simulink model "SIMULINK_PID_Tracking"  (R2023b)
settings: Solver=FixedStepAuto  StartTime=0.0  StopTime=sim_end_time  FixedStep=fixed_step_size  RelTol=1e-3
undefined symbols (not defined in the file): a, act_end, b, battery_threshold, bb, draw_gif, droneyeeUAV2_NUM, droneyeeUAV3_NUM, droneyeeUAV4_NUM, droneyeeUAV5_NUM, fixed_step_size, k, KD_x, KD_y, kd_z, KDD_x, KDD_y, KI_x, KI_y, ki_z, KII_x, KII_y, KP_x, KP_y, kp_z, KPP_x, KPP_y, lmt, omega, R, sim_end_time, uav10num, uav1num, uav2num, uav3num, uav4num, uav5num, uav6num, uav7num, uav8num, uav9num, UAV_NUM, Vel_Switch_1, Vel_Switch_10, Vel_Switch_11, Vel_Switch_12, Vel_Switch_13, Vel_Switch_14, Vel_Switch_15, Vel_Switch_16, Vel_Switch_17, Vel_Switch_18, Vel_Switch_19, Vel_Switch_2, Vel_Switch_20, Vel_Switch_3, Vel_Switch_4, Vel_Switch_5, Vel_Switch_6, Vel_Switch_7 ... (+12)
libraries: simulink x120, aerolibanimutils x1
(part 6 of 10)

== system SIMULINK_PID_Tracking/send_ctrl_signal_UAV/Send Command 2 ==
  pos : Inport
  u : Inport  Port=2
  Bus Selector : BusSelector  OutputSignals=droneyeeUAV2_states.x,droneyeeUAV2_states.y  OutputAsBus=on
  Bus Selector1 : BusSelector  OutputSignals=uav2.u_vx,uav2.u_vy,uav2.u_vz,uav2.u_rate_roll,uav2.u_rate_pitch,uav2.u_rate_yaw
  Clock : Clock
  Compare To Constant : simulink/Logic and Bit Operations/Compare To Constant  relop=>=  const=0.1  OutDataTypeStr=boolean
  Constant : Constant  Value=sim_end_time
  Constant1 : Constant  Value=0
  Constant2 : Constant  Value=droneyeeUAV2_NUM
  Constant3 : Constant  Value=Vel_Switch_2
  Constant4 : Constant  Value=0
  K : Gain
  K1 : Gain
  K2 : Gain
  Logical Operator : Logic  Inputs=3  AllPortsSameDT=off  OutDataTypeStr=boolean
  Mux : Mux  Inputs=8
  Mux1 : Mux  Inputs=5
  Subsystem : Subsystem
  Sum : Sum  Inputs=|-+
  Switch{1..3,6,12} (5 alike) : Switch  Criteria=u2 > Threshold  Threshold=0.001  SaturateOnIntegerOverflow=off  InputSameDT=off
  Switch4 : Switch  Criteria=u2 > Threshold  SaturateOnIntegerOverflow=off  InputSameDT=off
  Switch5 : Switch  Criteria=u2 > Threshold  SaturateOnIntegerOverflow=off  InputSameDT=off
  uav2 : Constant
  tag scope: copterSend2=global, sim_CopterSend2=global
  wires:
  Constant1/1 -> Switch3/3, Switch2/3, Switch1/3, Switch12/3
  Switch1/1 -> K/1
  Bus Selector1/2 -> Switch1/1  "<u_vy>"
  Switch2/1 -> K2/1
  Bus Selector1/3 -> Switch2/1  "<u_vz>"
  Switch3/1 -> K1/1
  Logical Operator/1 -> Switch1/2, Switch12/2, Switch2/2, Switch3/2
  Clock/1 -> Sum/1
  Constant/1 -> Sum/2
  Sum/1 -> Compare To Constant/1
  Compare To Constant/1 -> Logical Operator/2
  pos/1 -> Bus Selector/1
  Bus Selector/1 -> Subsystem/1(In1)
  u/1 -> Bus Selector1/1
  Bus Selector1/1 -> Switch12/1  "<u_vx>"
  Bus Selector1/6 -> Switch3/1  "<u_rate_yaw>"
  Bus Selector1/4 -> Mux/5  "<u_rate_roll>"
  Bus Selector1/5 -> Mux/6  "<u_rate_pitch>"
  Constant2/1 -> Mux/1
  Constant3/1 -> Logical Operator/3
  Switch6/1 -> Mux/8
  Subsystem/1(Out1) -> Logical Operator/1
  Switch4/1 -> [sim_CopterSend2]
  [sim_flag] -> Switch5/2, Switch4/2
  Switch5/1 -> [copterSend2]
  Mux/1 -> Switch5/1
  Mux1/1 -> Switch4/3
  K/1 -> Mux1/3, Mux/3
  K1/1 -> Mux1/5, Mux/7
  K2/1 -> Mux1/4, Mux/4
  Switch12/1 -> Mux1/2, Mux/2
  Constant4/1 -> Mux1/1
  uav2/1 -> Switch6/3
  [mode1] -> Switch6/2, Switch6/1

== system SIMULINK_PID_Tracking/send_ctrl_signal_UAV/Send Command 3 ==
  pos : Inport
  u : Inport  Port=2
  Bus Selector : BusSelector  OutputSignals=droneyeeUAV3_states.x,droneyeeUAV3_states.y  OutputAsBus=on
  Bus Selector1 : BusSelector  OutputSignals=uav3.u_vx,uav3.u_vy,uav3.u_vz,uav3.u_rate_roll,uav3.u_rate_pitch,uav3.u_rate_yaw
  Clock : Clock
  Compare To Constant : simulink/Logic and Bit Operations/Compare To Constant  relop=>=  const=0.1  OutDataTypeStr=boolean
  Constant : Constant  Value=sim_end_time
  Constant1 : Constant  Value=0
  Constant2 : Constant  Value=droneyeeUAV3_NUM
  Constant3 : Constant  Value=Vel_Switch_3
  Constant4 : Constant  Value=0
  K : Gain
  K1 : Gain
  K2 : Gain
  Logical Operator : Logic  Inputs=3  AllPortsSameDT=off  OutDataTypeStr=boolean
  Mux : Mux  Inputs=8
  Mux1 : Mux  Inputs=5
  Subsystem : Subsystem
  Sum : Sum  Inputs=|-+
  Switch{1..3,6,12} (5 alike) : Switch  Criteria=u2 > Threshold  Threshold=0.001  SaturateOnIntegerOverflow=off  InputSameDT=off
  Switch4 : Switch  Criteria=u2 > Threshold  SaturateOnIntegerOverflow=off  InputSameDT=off
  Switch5 : Switch  Criteria=u2 > Threshold  SaturateOnIntegerOverflow=off  InputSameDT=off
  uav3 : Constant
  tag scope: copterSend3=global, sim_CopterSend3=global
  wires:
  Constant1/1 -> Switch3/3, Switch2/3, Switch1/3, Switch12/3
  Switch1/1 -> K/1
  Bus Selector1/2 -> Switch1/1  "<u_vy>"
  Switch2/1 -> K2/1
  Bus Selector1/3 -> Switch2/1  "<u_vz>"
  Switch3/1 -> K1/1
  Logical Operator/1 -> Switch1/2, Switch12/2, Switch2/2, Switch3/2
  Clock/1 -> Sum/1
  Constant/1 -> Sum/2
  Sum/1 -> Compare To Constant/1
  Compare To Constant/1 -> Logical Operator/2
  pos/1 -> Bus Selector/1
  Bus Selector/1 -> Subsystem/1(In1)
  u/1 -> Bus Selector1/1
  Bus Selector1/1 -> Switch12/1  "<u_vx>"
  Bus Selector1/6 -> Switch3/1  "<u_rate_yaw>"
  Bus Selector1/4 -> Mux/5  "<u_rate_roll>"
  Bus Selector1/5 -> Mux/6  "<u_rate_pitch>"
  Constant2/1 -> Mux/1
  Constant3/1 -> Logical Operator/3
  Switch6/1 -> Mux/8
  Subsystem/1(Out1) -> Logical Operator/1
  Switch4/1 -> [sim_CopterSend3]
  [sim_flag] -> Switch5/2, Switch4/2
  Switch5/1 -> [copterSend3]
  Mux/1 -> Switch5/1
  Mux1/1 -> Switch4/3
  K/1 -> Mux1/3, Mux/3
  K1/1 -> Mux1/5, Mux/7
  K2/1 -> Mux1/4, Mux/4
  Switch12/1 -> Mux1/2, Mux/2
  Constant4/1 -> Mux1/1
  uav3/1 -> Switch6/3
  [mode1] -> Switch6/2, Switch6/1

== system SIMULINK_PID_Tracking/send_ctrl_signal_UAV/Send Command 4 ==
  pos : Inport
  u : Inport  Port=2
  Bus Selector : BusSelector  OutputSignals=droneyeeUAV4_states.x,droneyeeUAV4_states.y  OutputAsBus=on
  Bus Selector1 : BusSelector  OutputSignals=uav4.u_vx,uav4.u_vy,uav4.u_vz,uav4.u_rate_roll,uav4.u_rate_pitch,uav4.u_rate_yaw
  Clock : Clock
  Compare To Constant : simulink/Logic and Bit Operations/Compare To Constant  relop=>=  const=0.1  OutDataTypeStr=boolean
  Constant : Constant  Value=sim_end_time
  Constant1 : Constant  Value=0
  Constant2 : Constant  Value=droneyeeUAV4_NUM
  Constant3 : Constant  Value=Vel_Switch_4
  Constant4 : Constant  Value=0
  K : Gain
  K1 : Gain
  K2 : Gain
  Logical Operator : Logic  Inputs=3  AllPortsSameDT=off  OutDataTypeStr=boolean
  Mux : Mux  Inputs=8
  Mux1 : Mux  Inputs=5
  Subsystem : Subsystem
  Sum : Sum  Inputs=|-+
  Switch{1..3,6,12} (5 alike) : Switch  Criteria=u2 > Threshold  Threshold=0.001  SaturateOnIntegerOverflow=off  InputSameDT=off
  Switch4 : Switch  Criteria=u2 > Threshold  SaturateOnIntegerOverflow=off  InputSameDT=off
  Switch5 : Switch  Criteria=u2 > Threshold  SaturateOnIntegerOverflow=off  InputSameDT=off
  uav4 : Constant
  tag scope: copterSend4=global, sim_CopterSend4=global
  wires:
  Constant1/1 -> Switch3/3, Switch2/3, Switch1/3, Switch12/3
  Switch1/1 -> K/1
  Bus Selector1/2 -> Switch1/1  "<u_vy>"
  Switch2/1 -> K2/1
  Bus Selector1/3 -> Switch2/1  "<u_vz>"
  Switch3/1 -> K1/1
  Logical Operator/1 -> Switch1/2, Switch12/2, Switch2/2, Switch3/2
  Clock/1 -> Sum/1
  Constant/1 -> Sum/2
  Sum/1 -> Compare To Constant/1
  Compare To Constant/1 -> Logical Operator/2
  pos/1 -> Bus Selector/1
  u/1 -> Bus Selector1/1
  Bus Selector1/1 -> Switch12/1  "<u_vx>"
  Bus Selector1/6 -> Switch3/1  "<u_rate_yaw>"
  Bus Selector1/4 -> Mux/5  "<u_rate_roll>"
  Bus Selector1/5 -> Mux/6  "<u_rate_pitch>"
  Constant2/1 -> Mux/1
  Constant3/1 -> Logical Operator/3
  Switch6/1 -> Mux/8
  Bus Selector/1 -> Subsystem/1(In1)
  Subsystem/1(Out1) -> Logical Operator/1
  Switch4/1 -> [sim_CopterSend4]
  [sim_flag] -> Switch5/2, Switch4/2
  Switch5/1 -> [copterSend4]
  Mux/1 -> Switch5/1
  Mux1/1 -> Switch4/3
  K/1 -> Mux1/3, Mux/3
  K1/1 -> Mux1/5, Mux/7
  K2/1 -> Mux1/4, Mux/4
  Switch12/1 -> Mux1/2, Mux/2
  Constant4/1 -> Mux1/1
  uav4/1 -> Switch6/3
  [mode1] -> Switch6/2, Switch6/1

== system SIMULINK_PID_Tracking/send_ctrl_signal_UAV/Send Command 5 ==
  pos : Inport
  u : Inport  Port=2
  Bus Selector : BusSelector  OutputSignals=x,y  OutputAsBus=on
  Bus Selector1 : BusSelector  OutputSignals=u_vx,u_vy,u_vz,u_rate_roll,u_rate_pitch,u_rate_yaw
  Clock : Clock
  Compare To Constant : simulink/Logic and Bit Operations/Compare To Constant  relop=>=  const=0.1  OutDataTypeStr=boolean
  Constant : Constant  Value=sim_end_time
  Constant1 : Constant  Value=0
  Constant2 : Constant  Value=droneyeeUAV5_NUM
  Constant3 : Constant  Value=Vel_Switch_5
  Constant4 : Constant  Value=0
  K : Gain
  K1 : Gain
  K2 : Gain
  Logical Operator : Logic  Inputs=3  AllPortsSameDT=off  OutDataTypeStr=boolean
  Mux : Mux  Inputs=8
  Mux1 : Mux  Inputs=5
  Subsystem : Subsystem
  Sum : Sum  Inputs=|-+
  Switch{1..3,6,12} (5 alike) : Switch  Criteria=u2 > Threshold  Threshold=0.001  SaturateOnIntegerOverflow=off  InputSameDT=off
  Switch4 : Switch  Criteria=u2 > Threshold  SaturateOnIntegerOverflow=off  InputSameDT=off
  Switch5 : Switch  Criteria=u2 > Threshold  SaturateOnIntegerOverflow=off  InputSameDT=off
  uav5 : Constant
  tag scope: copterSend5=global, sim_CopterSend5=global
  wires:
  Constant1/1 -> Switch3/3, Switch2/3, Switch1/3, Switch12/3
  Switch1/1 -> K/1
  Bus Selector1/2 -> Switch1/1  "<u_vy>"
  Switch2/1 -> K2/1
  Bus Selector1/3 -> Switch2/1  "<u_vz>"
  Switch3/1 -> K1/1
  Logical Operator/1 -> Switch1/2, Switch12/2, Switch2/2, Switch3/2
  Clock/1 -> Sum/1
  Constant/1 -> Sum/2
  Sum/1 -> Compare To Constant/1
  Compare To Constant/1 -> Logical Operator/2
  pos/1 -> Bus Selector/1
  Bus Selector/1 -> Subsystem/1(In1)
  u/1 -> Bus Selector1/1
  Bus Selector1/1 -> Switch12/1  "<u_vx>"
  Bus Selector1/6 -> Switch3/1  "<u_rate_yaw>"
  Bus Selector1/4 -> Mux/5  "<u_rate_roll>"
  Bus Selector1/5 -> Mux/6  "<u_rate_pitch>"
  Subsystem/1(Out1) -> Logical Operator/1
  Constant2/1 -> Mux/1
  Constant3/1 -> Logical Operator/3
  Switch6/1 -> Mux/8
  Switch4/1 -> [sim_CopterSend5]
  [sim_flag] -> Switch5/2, Switch4/2
  Switch5/1 -> [copterSend5]
  Mux/1 -> Switch5/1
  Mux1/1 -> Switch4/3
  K/1 -> Mux1/3, Mux/3
  K1/1 -> Mux1/5, Mux/7
  K2/1 -> Mux1/4, Mux/4
  Switch12/1 -> Mux1/2, Mux/2
  Constant4/1 -> Mux1/1
  uav5/1 -> Switch6/3
  [mode1] -> Switch6/2, Switch6/1

== system SIMULINK_PID_Tracking/send_ctrl_signal_UAV/Send Command 6 ==
  pos : Inport
  u : Inport  Port=2
  Bus Selector : BusSelector  OutputSignals=x,y  OutputAsBus=on
  Bus Selector1 : BusSelector  OutputSignals=u_vx,u_vy,u_vz,u_rate_roll,u_rate_pitch,u_rate_yaw
  Clock : Clock
  Compare To Constant : simulink/Logic and Bit Operations/Compare To Constant  relop=>=  const=0.1  OutDataTypeStr=boolean
  Constant : Constant  Value=sim_end_time
  Constant1 : Constant  Value=0
  Constant2 : Constant  Value=uav6num
  Constant3 : Constant  Value=Vel_Switch_6
  Constant4 : Constant  Value=0
  K : Gain
  K1 : Gain
  K2 : Gain
  Logical Operator : Logic  Inputs=3  AllPortsSameDT=off  OutDataTypeStr=boolean
  Mux : Mux  Inputs=8
  Mux1 : Mux  Inputs=5
  Subsystem : Subsystem
  Sum : Sum  Inputs=|-+
  Switch{1..3,6,12} (5 alike) : Switch  Criteria=u2 > Threshold  Threshold=0.001  SaturateOnIntegerOverflow=off  InputSameDT=off
  Switch4 : Switch  Criteria=u2 > Threshold  SaturateOnIntegerOverflow=off  InputSameDT=off
  Switch5 : Switch  Criteria=u2 > Threshold  SaturateOnIntegerOverflow=off  InputSameDT=off
  uav6 : Constant  Value=0
  tag scope: copterSend6=global, sim_CopterSend6=global
  wires:
  Constant1/1 -> Switch3/3, Switch2/3, Switch1/3, Switch12/3
  K1/1 -> Mux1/5, Mux/7
  Switch1/1 -> K/1
  Bus Selector1/2 -> Switch1/1  "<u_vy>"
  Switch2/1 -> K2/1
  Bus Selector1/3 -> Switch2/1  "<u_vz>"
  Switch3/1 -> K1/1
  Logical Operator/1 -> Switch1/2, Switch12/2, Switch2/2, Switch3/2
  K2/1 -> Mux1/4, Mux/4
  Clock/1 -> Sum/1
  Constant/1 -> Sum/2
  Sum/1 -> Compare To Constant/1
  Compare To Constant/1 -> Logical Operator/2
  pos/1 -> Bus Selector/1
  Bus Selector/1 -> Subsystem/1(In1)
  u/1 -> Bus Selector1/1
  Bus Selector1/1 -> Switch12/1  "<u_vx>"
  Bus Selector1/6 -> Switch3/1  "<u_rate_yaw>"
  Bus Selector1/4 -> Mux/5  "<u_rate_roll>"
  Bus Selector1/5 -> Mux/6  "<u_rate_pitch>"
  Constant2/1 -> Mux/1
  Constant3/1 -> Logical Operator/3
  Switch12/1 -> Mux1/2, Mux/2
  K/1 -> Mux1/3, Mux/3
  Switch6/1 -> Mux/8
  Subsystem/1(Out1) -> Logical Operator/1
  Constant4/1 -> Mux1/1
  Switch4/1 -> [sim_CopterSend6]
  Mux1/1 -> Switch4/3
  Mux/1 -> Switch5/1
  Switch5/1 -> [copterSend6]
  [sim_flag] -> Switch5/2, Switch4/2
  uav6/1 -> Switch6/3
  [mode1] -> Switch6/2, Switch6/1

== system SIMULINK_PID_Tracking/send_ctrl_signal_UAV/Send Command 7 ==
  pos : Inport
  u : Inport  Port=2
  Bus Selector : BusSelector  OutputSignals=x,y  OutputAsBus=on
  Bus Selector1 : BusSelector  OutputSignals=u_vx,u_vy,u_vz,u_rate_roll,u_rate_pitch,u_rate_yaw
  Clock : Clock
  Compare To Constant : simulink/Logic and Bit Operations/Compare To Constant  relop=>=  const=0.1  OutDataTypeStr=boolean
  Constant : Constant  Value=sim_end_time
  Constant1 : Constant  Value=0
  Constant2 : Constant  Value=uav7num
  Constant3 : Constant  Value=Vel_Switch_7
  Constant4 : Constant  Value=0
  K : Gain
  K1 : Gain
  K2 : Gain
  Logical Operator : Logic  Inputs=3  AllPortsSameDT=off  OutDataTypeStr=boolean
  Mux : Mux  Inputs=8
  Mux1 : Mux  Inputs=5
  Subsystem : Subsystem
  Sum : Sum  Inputs=|-+
  Switch{1..3,6,12} (5 alike) : Switch  Criteria=u2 > Threshold  Threshold=0.001  SaturateOnIntegerOverflow=off  InputSameDT=off
  Switch4 : Switch  Criteria=u2 > Threshold  SaturateOnIntegerOverflow=off  InputSameDT=off
  Switch5 : Switch  Criteria=u2 > Threshold  SaturateOnIntegerOverflow=off  InputSameDT=off
  uav7 : Constant  Value=0
  tag scope: copterSend7=global, sim_CopterSend7=global
  wires:
  Constant1/1 -> Switch3/3, Switch2/3, Switch1/3, Switch12/3
  K1/1 -> Mux1/5, Mux/7
  Switch1/1 -> K/1
  Bus Selector1/2 -> Switch1/1  "<u_vy>"
  Switch2/1 -> K2/1
  Bus Selector1/3 -> Switch2/1  "<u_vz>"
  Switch3/1 -> K1/1
  Logical Operator/1 -> Switch1/2, Switch12/2, Switch2/2, Switch3/2
  K2/1 -> Mux1/4, Mux/4
  Clock/1 -> Sum/1
  Constant/1 -> Sum/2
  Sum/1 -> Compare To Constant/1
  Compare To Constant/1 -> Logical Operator/2
  pos/1 -> Bus Selector/1
  Bus Selector/1 -> Subsystem/1(In1)
  u/1 -> Bus Selector1/1
  Bus Selector1/1 -> Switch12/1  "<u_vx>"
  Bus Selector1/6 -> Switch3/1  "<u_rate_yaw>"
  Bus Selector1/4 -> Mux/5  "<u_rate_roll>"
  Bus Selector1/5 -> Mux/6  "<u_rate_pitch>"
  Constant2/1 -> Mux/1
  Constant3/1 -> Logical Operator/3
  Switch12/1 -> Mux1/2, Mux/2
  K/1 -> Mux1/3, Mux/3
  Switch6/1 -> Mux/8
  Subsystem/1(Out1) -> Logical Operator/1
  Constant4/1 -> Mux1/1
  Switch4/1 -> [sim_CopterSend7]
  Mux1/1 -> Switch4/3
  Mux/1 -> Switch5/1
  Switch5/1 -> [copterSend7]
  [sim_flag] -> Switch5/2, Switch4/2
  uav7/1 -> Switch6/3
  [mode1] -> Switch6/2, Switch6/1

== system SIMULINK_PID_Tracking/send_ctrl_signal_UAV/Send Command 8 ==
  pos : Inport
  u : Inport  Port=2
  Bus Selector : BusSelector  OutputSignals=x,y  OutputAsBus=on
  Bus Selector1 : BusSelector  OutputSignals=u_vx,u_vy,u_vz,u_rate_roll,u_rate_pitch,u_rate_yaw
  Clock : Clock
  Compare To Constant : simulink/Logic and Bit Operations/Compare To Constant  relop=>=  const=0.1  OutDataTypeStr=boolean
  Constant : Constant  Value=sim_end_time
  Constant1 : Constant  Value=0
  Constant2 : Constant  Value=uav8num
  Constant3 : Constant  Value=Vel_Switch_8
  Constant4 : Constant  Value=0
  K : Gain
  K1 : Gain
  K2 : Gain
  Logical Operator : Logic  Inputs=3  AllPortsSameDT=off  OutDataTypeStr=boolean
  Mux : Mux  Inputs=8
  Mux1 : Mux  Inputs=5
  Subsystem : Subsystem
  Sum : Sum  Inputs=|-+
  Switch{1..3,6,12} (5 alike) : Switch  Criteria=u2 > Threshold  Threshold=0.001  SaturateOnIntegerOverflow=off  InputSameDT=off
  Switch4 : Switch  Criteria=u2 > Threshold  SaturateOnIntegerOverflow=off  InputSameDT=off
  Switch5 : Switch  Criteria=u2 > Threshold  SaturateOnIntegerOverflow=off  InputSameDT=off
  uav8 : Constant
  tag scope: copterSend8=global, sim_CopterSend8=global
  wires:
  Constant1/1 -> Switch3/3, Switch2/3, Switch1/3, Switch12/3
  K1/1 -> Mux1/5, Mux/7
  Switch1/1 -> K/1
  Bus Selector1/2 -> Switch1/1  "<u_vy>"
  Switch2/1 -> K2/1
  Bus Selector1/3 -> Switch2/1  "<u_vz>"
  Switch3/1 -> K1/1
  Logical Operator/1 -> Switch1/2, Switch12/2, Switch2/2, Switch3/2
  K2/1 -> Mux1/4, Mux/4
  Clock/1 -> Sum/1
  Constant/1 -> Sum/2
  Sum/1 -> Compare To Constant/1
  Compare To Constant/1 -> Logical Operator/2
  pos/1 -> Bus Selector/1
  Bus Selector/1 -> Subsystem/1(In1)
  u/1 -> Bus Selector1/1
  Bus Selector1/1 -> Switch12/1  "<u_vx>"
  Bus Selector1/6 -> Switch3/1  "<u_rate_yaw>"
  Bus Selector1/4 -> Mux/5  "<u_rate_roll>"
  Bus Selector1/5 -> Mux/6  "<u_rate_pitch>"
  Constant2/1 -> Mux/1
  Constant3/1 -> Logical Operator/3
  Switch12/1 -> Mux1/2, Mux/2
  K/1 -> Mux1/3, Mux/3
  Switch6/1 -> Mux/8
  Subsystem/1(Out1) -> Logical Operator/1
  Constant4/1 -> Mux1/1
  Switch4/1 -> [sim_CopterSend8]
  Mux1/1 -> Switch4/3
  Mux/1 -> Switch5/1
  Switch5/1 -> [copterSend8]
  [sim_flag] -> Switch5/2, Switch4/2
  uav8/1 -> Switch6/3
  [mode1] -> Switch6/2, Switch6/1

== system SIMULINK_PID_Tracking/send_ctrl_signal_UAV/Send Command 9 ==
  pos : Inport
  u : Inport  Port=2
  Bus Selector : BusSelector  OutputSignals=x,y  OutputAsBus=on
  Bus Selector1 : BusSelector  OutputSignals=u_vx,u_vy,u_vz,u_rate_roll,u_rate_pitch,u_rate_yaw
  Clock : Clock
  Compare To Constant : simulink/Logic and Bit Operations/Compare To Constant  relop=>=  const=0.1  OutDataTypeStr=boolean
  Constant : Constant  Value=sim_end_time
  Constant1 : Constant  Value=0
  Constant2 : Constant  Value=uav9num
  Constant3 : Constant  Value=Vel_Switch_9
  Constant4 : Constant  Value=0
  K : Gain
  K1 : Gain
  K2 : Gain
  Logical Operator : Logic  Inputs=3  AllPortsSameDT=off  OutDataTypeStr=boolean
  Mux : Mux  Inputs=8
  Mux1 : Mux  Inputs=5
  Subsystem : Subsystem
  Sum : Sum  Inputs=|-+
  Switch{1..3,6,12} (5 alike) : Switch  Criteria=u2 > Threshold  Threshold=0.001  SaturateOnIntegerOverflow=off  InputSameDT=off
  Switch4 : Switch  Criteria=u2 > Threshold  SaturateOnIntegerOverflow=off  InputSameDT=off
  Switch5 : Switch  Criteria=u2 > Threshold  SaturateOnIntegerOverflow=off  InputSameDT=off
  uav9 : Constant
  tag scope: copterSend9=global, sim_CopterSend9=global
  wires:
  Constant1/1 -> Switch3/3, Switch2/3, Switch1/3, Switch12/3
  K1/1 -> Mux1/5, Mux/7
  Switch1/1 -> K/1
  Bus Selector1/2 -> Switch1/1  "<u_vy>"
  Switch2/1 -> K2/1
  Bus Selector1/3 -> Switch2/1  "<u_vz>"
  Switch3/1 -> K1/1
  Logical Operator/1 -> Switch1/2, Switch12/2, Switch2/2, Switch3/2
  K2/1 -> Mux1/4, Mux/4
  Clock/1 -> Sum/1
  Constant/1 -> Sum/2
  Sum/1 -> Compare To Constant/1
  Compare To Constant/1 -> Logical Operator/2
  pos/1 -> Bus Selector/1
  Bus Selector/1 -> Subsystem/1(In1)
  u/1 -> Bus Selector1/1
  Bus Selector1/1 -> Switch12/1  "<u_vx>"
  Bus Selector1/6 -> Switch3/1  "<u_rate_yaw>"
  Bus Selector1/4 -> Mux/5  "<u_rate_roll>"
  Bus Selector1/5 -> Mux/6  "<u_rate_pitch>"
  Constant2/1 -> Mux/1
  Constant3/1 -> Logical Operator/3
  Switch12/1 -> Mux1/2, Mux/2
  K/1 -> Mux1/3, Mux/3
  Switch6/1 -> Mux/8
  Subsystem/1(Out1) -> Logical Operator/1
  Constant4/1 -> Mux1/1
  Switch4/1 -> [sim_CopterSend9]
  Mux1/1 -> Switch4/3
  Mux/1 -> Switch5/1
  Switch5/1 -> [copterSend9]
  [sim_flag] -> Switch5/2, Switch4/2
  uav9/1 -> Switch6/3
  [mode1] -> Switch6/2, Switch6/1

== system SIMULINK_PID_Tracking/send_ctrl_signal_UAV/Subsystem ==
  states_d : Inport
  ctrl : Inport  Port=2
  Bus Selector : BusSelector  OutputSignals=states1_2_d,states_3_4_d,states_5_6_d,states_7_8_d,states_9_10_d
  Bus Selector1 : BusSelector  OutputSignals=droneyeeUAV1_states,droneyeeUAV2_states  OutputAsBus=on
  Bus Selector2 : BusSelector  OutputSignals=ctrl_1_2,ctrl_3_4,ctrl_5_6,ctrl_7_8,ctrl_9_10
  Bus Selector5 : BusSelector  OutputSignals=droneyeeUAV9_states,droneyeeUAV10_states  OutputAsBus=on
  Bus Selector6 : BusSelector  OutputSignals=droneyeeUAV3_states,droneyeeUAV4_states  OutputAsBus=on
  Bus Selector7 : BusSelector  OutputSignals=droneyeeUAV5_states,droneyeeUAV6_states  OutputAsBus=on
  Bus Selector8 : BusSelector  OutputSignals=droneyeeUAV7_states,droneyeeUAV8_states  OutputAsBus=on
  logger_UAV : Subsystem
  wires:
  Bus Selector/1 -> logger_UAV/6(state_d1_2)  "<states1_2_d>"
  Bus Selector/2 -> logger_UAV/7(state_d3_4)  "<states_3_4_d>"
  [uav_states] -> Bus Selector8/1, Bus Selector7/1, Bus Selector6/1, Bus Selector1/1, Bus Selector5/1
  Bus Selector1/1 -> logger_UAV/1(state1_2)
  Bus Selector6/1 -> logger_UAV/2(state3_4)
  Bus Selector2/2 -> logger_UAV/12(u3_4)  "<ctrl_3_4>"
  Bus Selector2/1 -> logger_UAV/11(u1_2)  "<ctrl_1_2>"
  Bus Selector7/1 -> logger_UAV/3(state5_6)
  Bus Selector2/3 -> logger_UAV/13(u5_6)  "<ctrl_5_6>"
  states_d/1 -> Bus Selector/1
  ctrl/1 -> Bus Selector2/1
  Bus Selector/3 -> logger_UAV/8(state_d5_6)  "<states_5_6_d>"
  Bus Selector8/1 -> logger_UAV/4(state7_8)
  Bus Selector5/1 -> logger_UAV/5(In5)
  Bus Selector/4 -> logger_UAV/9(In9)  "<states_7_8_d>"
  Bus Selector/5 -> logger_UAV/10(In10)  "<states_9_10_d>"
  Bus Selector2/4 -> logger_UAV/14(In14)  "<ctrl_7_8>"
  Bus Selector2/5 -> logger_UAV/15(In15)  "<ctrl_9_10>"

== system SIMULINK_PID_Tracking/send_ctrl_signal_car1/Send Command 1 ==
  pos : Inport
  u : Inport  Port=2
  Bus Selector : BusSelector  OutputSignals=droneyeeCAR1_states.x,droneyeeCAR1_states.y  OutputAsBus=on
  Bus Selector1 : BusSelector  OutputSignals=CAR1.u_vx,CAR1.u_vy,CAR1.u_vz,CAR1.u_rate_roll,CAR1.u_rate_pitch,CAR1.u_rate_yaw
  Clock : Clock
  Compare To Constant : simulink/Logic and Bit Operations/Compare To Constant  relop=>=  const=0.1  OutDataTypeStr=boolean
  Constant : Constant  Value=sim_end_time
  Constant1 : Constant  Value=0
  Constant2 : Constant  Value=uav1num
  Constant3 : Constant  Value=Vel_Switch_11
  Constant4 : Constant  Value=0
  K : Gain
  K1 : Gain
  K2 : Gain
  Logical Operator : Logic  Inputs=3  AllPortsSameDT=off  OutDataTypeStr=boolean
  Mux : Mux  Inputs=8
  Mux1 : Mux  Inputs=5
  Subsystem : Subsystem
  Sum : Sum  Inputs=|-+
  Switch{1..3,6,12} (5 alike) : Switch  Criteria=u2 > Threshold  Threshold=0.001  SaturateOnIntegerOverflow=off  InputSameDT=off
  Switch4 : Switch  Criteria=u2 > Threshold  SaturateOnIntegerOverflow=off  InputSameDT=off
  Switch5 : Switch  Criteria=u2 > Threshold  SaturateOnIntegerOverflow=off  InputSameDT=off
  uav1 : Constant  Value=0
  tag scope: carSend1=global, sim_CarSend1=global
  wires:
  Constant1/1 -> Switch3/3, Switch2/3, Switch1/3, Switch12/3
  K1/1 -> Mux1/5, Mux/7
  Switch1/1 -> K/1
  Bus Selector1/2 -> Switch1/1  "<u_vy>"
  Switch2/1 -> K2/1
  Bus Selector1/3 -> Switch2/1  "<u_vz>"
  Switch3/1 -> K1/1
  Logical Operator/1 -> Switch1/2, Switch12/2, Switch2/2, Switch3/2
  K2/1 -> Mux1/4, Mux/4
  Clock/1 -> Sum/1
  Constant/1 -> Sum/2
  Sum/1 -> Compare To Constant/1
  Compare To Constant/1 -> Logical Operator/2
  pos/1 -> Bus Selector/1
  Bus Selector/1 -> Subsystem/1(In1)
  u/1 -> Bus Selector1/1
  Bus Selector1/1 -> Switch12/1  "<u_vx>"
  Bus Selector1/6 -> Switch3/1  "<u_rate_yaw>"
  Bus Selector1/4 -> Mux/5  "<u_rate_roll>"
  Bus Selector1/5 -> Mux/6  "<u_rate_pitch>"
  Constant2/1 -> Mux/1
  Constant3/1 -> Logical Operator/3
  Switch12/1 -> Mux1/2, Mux/2
  K/1 -> Mux1/3, Mux/3
  Switch6/1 -> Mux/8
  Subsystem/1(Out1) -> Logical Operator/1
  Constant4/1 -> Mux1/1
  Switch4/1 -> [sim_CarSend1]
  Mux1/1 -> Switch4/3
  Mux/1 -> Switch5/1
  Switch5/1 -> [carSend1]
  [sim_flag] -> Switch5/2, Switch4/2
  uav1/1 -> Switch6/3
  [mode1] -> Switch6/2, Switch6/1

== system SIMULINK_PID_Tracking/send_ctrl_signal_car1/Send Command 10 ==
  pos : Inport
  u : Inport  Port=2
  Bus Selector : BusSelector  OutputSignals=x,y  OutputAsBus=on
  Bus Selector1 : BusSelector  OutputSignals=u_vx,u_vy,u_vz,u_rate_roll,u_rate_pitch,u_rate_yaw
  Clock : Clock
  Compare To Constant : simulink/Logic and Bit Operations/Compare To Constant  relop=>=  const=0.1  OutDataTypeStr=boolean
  Constant : Constant  Value=sim_end_time
  Constant1 : Constant  Value=0
  Constant2 : Constant  Value=uav10num
  Constant3 : Constant  Value=Vel_Switch_20
  Constant4 : Constant  Value=0
  K : Gain
  K1 : Gain
  K2 : Gain
  Logical Operator : Logic  Inputs=3  AllPortsSameDT=off  OutDataTypeStr=boolean
  Mux : Mux  Inputs=8
  Mux1 : Mux  Inputs=5
  Subsystem : Subsystem
  Sum : Sum  Inputs=|-+
  Switch{1..3,6,12} (5 alike) : Switch  Criteria=u2 > Threshold  Threshold=0.001  SaturateOnIntegerOverflow=off  InputSameDT=off
  Switch4 : Switch  Criteria=u2 > Threshold  SaturateOnIntegerOverflow=off  InputSameDT=off
  Switch5 : Switch  Criteria=u2 > Threshold  SaturateOnIntegerOverflow=off  InputSameDT=off
  uav10 : Constant
  tag scope: carSend10=global, sim_CarSend10=global
  wires:
  Constant1/1 -> Switch3/3, Switch2/3, Switch1/3, Switch12/3
  K1/1 -> Mux1/5, Mux/7
  Switch1/1 -> K/1
  Bus Selector1/2 -> Switch1/1  "<u_vy>"
  Switch2/1 -> K2/1
  Bus Selector1/3 -> Switch2/1  "<u_vz>"
  Switch3/1 -> K1/1
  Logical Operator/1 -> Switch1/2, Switch12/2, Switch2/2, Switch3/2
  K2/1 -> Mux1/4, Mux/4
  Clock/1 -> Sum/1
  Constant/1 -> Sum/2
  Sum/1 -> Compare To Constant/1
  Compare To Constant/1 -> Logical Operator/2
  pos/1 -> Bus Selector/1
  Bus Selector/1 -> Subsystem/1(In1)
  u/1 -> Bus Selector1/1
  Bus Selector1/1 -> Switch12/1  "<u_vx>"
  Bus Selector1/6 -> Switch3/1  "<u_rate_yaw>"
  Bus Selector1/4 -> Mux/5  "<u_rate_roll>"
  Bus Selector1/5 -> Mux/6  "<u_rate_pitch>"
  Constant2/1 -> Mux/1
  Constant3/1 -> Logical Operator/3
  Switch12/1 -> Mux1/2, Mux/2
  K/1 -> Mux1/3, Mux/3
  Switch6/1 -> Mux/8
  Subsystem/1(Out1) -> Logical Operator/1
  Constant4/1 -> Mux1/1
  Switch4/1 -> [sim_CarSend10]
  Mux1/1 -> Switch4/3
  Mux/1 -> Switch5/1
  Switch5/1 -> [carSend10]
  [sim_flag] -> Switch5/2, Switch4/2
  uav10/1 -> Switch6/3
  [mode1] -> Switch6/2, Switch6/1

== system SIMULINK_PID_Tracking/send_ctrl_signal_car1/Send Command 2 ==
  pos : Inport
  u : Inport  Port=2
  Bus Selector : BusSelector  OutputSignals=droneyeeCAR2_states.x,droneyeeCAR2_states.y  OutputAsBus=on
  Bus Selector1 : BusSelector  OutputSignals=CAR2.u_vx,CAR2.u_vy,CAR2.u_vz,CAR2.u_rate_roll,CAR2.u_rate_pitch,CAR2.u_rate_yaw
  Clock : Clock
  Compare To Constant : simulink/Logic and Bit Operations/Compare To Constant  relop=>=  const=0.1  OutDataTypeStr=boolean
  Constant : Constant  Value=sim_end_time
  Constant1 : Constant  Value=0
  Constant2 : Constant  Value=droneyeeUAV2_NUM
  Constant3 : Constant  Value=Vel_Switch_12
  Constant4 : Constant  Value=0
  K : Gain
  K1 : Gain
  K2 : Gain
  Logical Operator : Logic  Inputs=3  AllPortsSameDT=off  OutDataTypeStr=boolean
  Mux : Mux  Inputs=8
  Mux1 : Mux  Inputs=5
  Subsystem : Subsystem
  Sum : Sum  Inputs=|-+
  Switch{1..3,6,12} (5 alike) : Switch  Criteria=u2 > Threshold  Threshold=0.001  SaturateOnIntegerOverflow=off  InputSameDT=off
  Switch4 : Switch  Criteria=u2 > Threshold  SaturateOnIntegerOverflow=off  InputSameDT=off
  Switch5 : Switch  Criteria=u2 > Threshold  SaturateOnIntegerOverflow=off  InputSameDT=off
  uav2 : Constant
  tag scope: carSend2=global, sim_CarSend2=global
  wires:
  Constant1/1 -> Switch3/3, Switch2/3, Switch1/3, Switch12/3
  Switch1/1 -> K/1
  Bus Selector1/2 -> Switch1/1  "<u_vy>"
  Switch2/1 -> K2/1
  Bus Selector1/3 -> Switch2/1  "<u_vz>"
  Switch3/1 -> K1/1
  Logical Operator/1 -> Switch1/2, Switch12/2, Switch2/2, Switch3/2
  Clock/1 -> Sum/1
  Constant/1 -> Sum/2
  Sum/1 -> Compare To Constant/1
  Compare To Constant/1 -> Logical Operator/2
  pos/1 -> Bus Selector/1
  Bus Selector/1 -> Subsystem/1(In1)
  u/1 -> Bus Selector1/1
  Bus Selector1/1 -> Switch12/1  "<u_vx>"
  Bus Selector1/6 -> Switch3/1  "<u_rate_yaw>"
  Bus Selector1/4 -> Mux/5  "<u_rate_roll>"
  Bus Selector1/5 -> Mux/6  "<u_rate_pitch>"
  Constant2/1 -> Mux/1
  Constant3/1 -> Logical Operator/3
  Switch6/1 -> Mux/8
  Subsystem/1(Out1) -> Logical Operator/1
  Switch4/1 -> [sim_CarSend2]
  [sim_flag] -> Switch5/2, Switch4/2
  Switch5/1 -> [carSend2]
  Mux/1 -> Switch5/1
  Mux1/1 -> Switch4/3
  K/1 -> Mux1/3, Mux/3
  K1/1 -> Mux1/5, Mux/7
  K2/1 -> Mux1/4, Mux/4
  Switch12/1 -> Mux1/2, Mux/2
  Constant4/1 -> Mux1/1
  uav2/1 -> Switch6/3
  [mode1] -> Switch6/2, Switch6/1

== system SIMULINK_PID_Tracking/send_ctrl_signal_car1/Send Command 3 ==
  pos : Inport
  u : Inport  Port=2
  Bus Selector : BusSelector  OutputSignals=droneyeeCAR3_states.x,droneyeeCAR3_states.y  OutputAsBus=on
  Bus Selector1 : BusSelector  OutputSignals=CAR3.u_vx,CAR3.u_vy,CAR3.u_vz,CAR3.u_rate_roll,CAR3.u_rate_pitch,CAR3.u_rate_yaw
  Clock : Clock
  Compare To Constant : simulink/Logic and Bit Operations/Compare To Constant  relop=>=  const=0.1  OutDataTypeStr=boolean
  Constant : Constant  Value=sim_end_time
  Constant1 : Constant  Value=0
  Constant2 : Constant  Value=droneyeeUAV3_NUM
  Constant3 : Constant  Value=Vel_Switch_13
  Constant4 : Constant  Value=0
  K : Gain
  K1 : Gain
  K2 : Gain
  Logical Operator : Logic  Inputs=3  AllPortsSameDT=off  OutDataTypeStr=boolean
  Mux : Mux  Inputs=8
  Mux1 : Mux  Inputs=5
  Subsystem : Subsystem
  Sum : Sum  Inputs=|-+
  Switch{1..3,6,12} (5 alike) : Switch  Criteria=u2 > Threshold  Threshold=0.001  SaturateOnIntegerOverflow=off  InputSameDT=off
  Switch4 : Switch  Criteria=u2 > Threshold  SaturateOnIntegerOverflow=off  InputSameDT=off
  Switch5 : Switch  Criteria=u2 > Threshold  SaturateOnIntegerOverflow=off  InputSameDT=off
  uav3 : Constant
  tag scope: carSend3=global, sim_CarSend3=global
  wires:
  Constant1/1 -> Switch3/3, Switch2/3, Switch1/3, Switch12/3
  Switch1/1 -> K/1
  Bus Selector1/2 -> Switch1/1  "<u_vy>"
  Switch2/1 -> K2/1
  Bus Selector1/3 -> Switch2/1  "<u_vz>"
  Switch3/1 -> K1/1
  Logical Operator/1 -> Switch1/2, Switch12/2, Switch2/2, Switch3/2
  Clock/1 -> Sum/1
  Constant/1 -> Sum/2
  Sum/1 -> Compare To Constant/1
  Compare To Constant/1 -> Logical Operator/2
  pos/1 -> Bus Selector/1
  Bus Selector/1 -> Subsystem/1(In1)
  u/1 -> Bus Selector1/1
  Bus Selector1/1 -> Switch12/1  "<u_vx>"
  Bus Selector1/6 -> Switch3/1  "<u_rate_yaw>"
  Bus Selector1/4 -> Mux/5  "<u_rate_roll>"
  Bus Selector1/5 -> Mux/6  "<u_rate_pitch>"
  Constant2/1 -> Mux/1
  Constant3/1 -> Logical Operator/3
  Switch6/1 -> Mux/8
  Subsystem/1(Out1) -> Logical Operator/1
  Switch4/1 -> [sim_CarSend3]
  [sim_flag] -> Switch5/2, Switch4/2
  Switch5/1 -> [carSend3]
  Mux/1 -> Switch5/1
  Mux1/1 -> Switch4/3
  K/1 -> Mux1/3, Mux/3
  K1/1 -> Mux1/5, Mux/7
  K2/1 -> Mux1/4, Mux/4
  Switch12/1 -> Mux1/2, Mux/2
  Constant4/1 -> Mux1/1
  uav3/1 -> Switch6/3
  [mode1] -> Switch6/2, Switch6/1

== system SIMULINK_PID_Tracking/send_ctrl_signal_car1/Send Command 4 ==
  pos : Inport
  u : Inport  Port=2
  Bus Selector : BusSelector  OutputSignals=droneyeeCAR4_states.x,droneyeeCAR4_states.y  OutputAsBus=on
  Bus Selector1 : BusSelector  OutputSignals=CAR4.u_vx,CAR4.u_vy,CAR4.u_vz,CAR4.u_rate_roll,CAR4.u_rate_pitch,CAR4.u_rate_yaw
  Clock : Clock
  Compare To Constant : simulink/Logic and Bit Operations/Compare To Constant  relop=>=  const=0.1  OutDataTypeStr=boolean
  Constant : Constant  Value=sim_end_time
  Constant1 : Constant  Value=0
  Constant2 : Constant  Value=droneyeeUAV4_NUM
  Constant3 : Constant  Value=Vel_Switch_14
  Constant4 : Constant  Value=0
  K : Gain
  K1 : Gain
  K2 : Gain
  Logical Operator : Logic  Inputs=3  AllPortsSameDT=off  OutDataTypeStr=boolean
  Mux : Mux  Inputs=8
  Mux1 : Mux  Inputs=5
  Subsystem : Subsystem
  Sum : Sum  Inputs=|-+
  Switch{1..3,6,12} (5 alike) : Switch  Criteria=u2 > Threshold  Threshold=0.001  SaturateOnIntegerOverflow=off  InputSameDT=off
  Switch4 : Switch  Criteria=u2 > Threshold  SaturateOnIntegerOverflow=off  InputSameDT=off
  Switch5 : Switch  Criteria=u2 > Threshold  SaturateOnIntegerOverflow=off  InputSameDT=off
  uav4 : Constant
  tag scope: carSend4=global, sim_CarSend4=global
  wires:
  Constant1/1 -> Switch3/3, Switch2/3, Switch1/3, Switch12/3
  Switch1/1 -> K/1
  Bus Selector1/2 -> Switch1/1  "<u_vy>"
  Switch2/1 -> K2/1
  Bus Selector1/3 -> Switch2/1  "<u_vz>"
  Switch3/1 -> K1/1
  Logical Operator/1 -> Switch1/2, Switch12/2, Switch2/2, Switch3/2
  Clock/1 -> Sum/1
  Constant/1 -> Sum/2
  Sum/1 -> Compare To Constant/1
  Compare To Constant/1 -> Logical Operator/2
  pos/1 -> Bus Selector/1
  u/1 -> Bus Selector1/1
  Bus Selector1/1 -> Switch12/1  "<u_vx>"
  Bus Selector1/6 -> Switch3/1  "<u_rate_yaw>"
  Bus Selector1/4 -> Mux/5  "<u_rate_roll>"
  Bus Selector1/5 -> Mux/6  "<u_rate_pitch>"
  Constant2/1 -> Mux/1
  Constant3/1 -> Logical Operator/3
  Switch6/1 -> Mux/8
  Bus Selector/1 -> Subsystem/1(In1)
  Subsystem/1(Out1) -> Logical Operator/1
  Switch4/1 -> [sim_CarSend4]
  [sim_flag] -> Switch5/2, Switch4/2
  Switch5/1 -> [carSend4]
  Mux/1 -> Switch5/1
  Mux1/1 -> Switch4/3
  K/1 -> Mux1/3, Mux/3
  K1/1 -> Mux1/5, Mux/7
  K2/1 -> Mux1/4, Mux/4
  Switch12/1 -> Mux1/2, Mux/2
  Constant4/1 -> Mux1/1
  uav4/1 -> Switch6/3
  [mode1] -> Switch6/2, Switch6/1

== system SIMULINK_PID_Tracking/send_ctrl_signal_car1/Send Command 5 ==
  pos : Inport
  u : Inport  Port=2
  Bus Selector : BusSelector  OutputSignals=x,y  OutputAsBus=on
  Bus Selector1 : BusSelector  OutputSignals=u_vx,u_vy,u_vz,u_rate_roll,u_rate_pitch,u_rate_yaw
  Clock : Clock
  Compare To Constant : simulink/Logic and Bit Operations/Compare To Constant  relop=>=  const=0.1  OutDataTypeStr=boolean
  Constant : Constant  Value=sim_end_time
  Constant1 : Constant  Value=0
  Constant2 : Constant  Value=droneyeeUAV5_NUM
  Constant3 : Constant  Value=Vel_Switch_15
  Constant4 : Constant  Value=0
  K : Gain
  K1 : Gain
  K2 : Gain
  Logical Operator : Logic  Inputs=3  AllPortsSameDT=off  OutDataTypeStr=boolean
  Mux : Mux  Inputs=8
  Mux1 : Mux  Inputs=5
  Subsystem : Subsystem
  Sum : Sum  Inputs=|-+
  Switch{1..3,6,12} (5 alike) : Switch  Criteria=u2 > Threshold  Threshold=0.001  SaturateOnIntegerOverflow=off  InputSameDT=off
  Switch4 : Switch  Criteria=u2 > Threshold  SaturateOnIntegerOverflow=off  InputSameDT=off
  Switch5 : Switch  Criteria=u2 > Threshold  SaturateOnIntegerOverflow=off  InputSameDT=off
  uav5 : Constant
  tag scope: carSend5=global, sim_CarSend5=global
  wires:
  Constant1/1 -> Switch3/3, Switch2/3, Switch1/3, Switch12/3
  Switch1/1 -> K/1
  Bus Selector1/2 -> Switch1/1  "<u_vy>"
  Switch2/1 -> K2/1
  Bus Selector1/3 -> Switch2/1  "<u_vz>"
  Switch3/1 -> K1/1
  Logical Operator/1 -> Switch1/2, Switch12/2, Switch2/2, Switch3/2
  Clock/1 -> Sum/1
  Constant/1 -> Sum/2
  Sum/1 -> Compare To Constant/1
  Compare To Constant/1 -> Logical Operator/2
  pos/1 -> Bus Selector/1
  Bus Selector/1 -> Subsystem/1(In1)
  u/1 -> Bus Selector1/1
  Bus Selector1/1 -> Switch12/1  "<u_vx>"
  Bus Selector1/6 -> Switch3/1  "<u_rate_yaw>"
  Bus Selector1/4 -> Mux/5  "<u_rate_roll>"
  Bus Selector1/5 -> Mux/6  "<u_rate_pitch>"
  Subsystem/1(Out1) -> Logical Operator/1
  Constant2/1 -> Mux/1
  Constant3/1 -> Logical Operator/3
  Switch6/1 -> Mux/8
  Switch4/1 -> [sim_CarSend5]
  [sim_flag] -> Switch5/2, Switch4/2
  Switch5/1 -> [carSend5]
  Mux/1 -> Switch5/1
  Mux1/1 -> Switch4/3
  K/1 -> Mux1/3, Mux/3
  K1/1 -> Mux1/5, Mux/7
  K2/1 -> Mux1/4, Mux/4
  Switch12/1 -> Mux1/2, Mux/2
  Constant4/1 -> Mux1/1
  uav5/1 -> Switch6/3
  [mode1] -> Switch6/2, Switch6/1

== system SIMULINK_PID_Tracking/send_ctrl_signal_car1/Send Command 6 ==
  pos : Inport
  u : Inport  Port=2
  Bus Selector : BusSelector  OutputSignals=x,y  OutputAsBus=on
  Bus Selector1 : BusSelector  OutputSignals=u_vx,u_vy,u_vz,u_rate_roll,u_rate_pitch,u_rate_yaw
  Clock : Clock
  Compare To Constant : simulink/Logic and Bit Operations/Compare To Constant  relop=>=  const=0.1  OutDataTypeStr=boolean
  Constant : Constant  Value=sim_end_time
  Constant1 : Constant  Value=0
  Constant2 : Constant  Value=uav6num
  Constant3 : Constant  Value=Vel_Switch_16
  Constant4 : Constant  Value=0
  K : Gain
  K1 : Gain
  K2 : Gain
  Logical Operator : Logic  Inputs=3  AllPortsSameDT=off  OutDataTypeStr=boolean
  Mux : Mux  Inputs=8
  Mux1 : Mux  Inputs=5
  Subsystem : Subsystem
  Sum : Sum  Inputs=|-+
  Switch{1..3,6,12} (5 alike) : Switch  Criteria=u2 > Threshold  Threshold=0.001  SaturateOnIntegerOverflow=off  InputSameDT=off
  Switch4 : Switch  Criteria=u2 > Threshold  SaturateOnIntegerOverflow=off  InputSameDT=off
  Switch5 : Switch  Criteria=u2 > Threshold  SaturateOnIntegerOverflow=off  InputSameDT=off
  uav6 : Constant  Value=3
  tag scope: carSend6=global, sim_CarSend6=global
  wires:
  Constant1/1 -> Switch3/3, Switch2/3, Switch1/3, Switch12/3
  K1/1 -> Mux1/5, Mux/7
  Switch1/1 -> K/1
  Bus Selector1/2 -> Switch1/1  "<u_vy>"
  Switch2/1 -> K2/1
  Bus Selector1/3 -> Switch2/1  "<u_vz>"
  Switch3/1 -> K1/1
  Logical Operator/1 -> Switch1/2, Switch12/2, Switch2/2, Switch3/2
  K2/1 -> Mux1/4, Mux/4
  Clock/1 -> Sum/1
  Constant/1 -> Sum/2
  Sum/1 -> Compare To Constant/1
  Compare To Constant/1 -> Logical Operator/2
  pos/1 -> Bus Selector/1
  Bus Selector/1 -> Subsystem/1(In1)
  u/1 -> Bus Selector1/1
  Bus Selector1/1 -> Switch12/1  "<u_vx>"
  Bus Selector1/6 -> Switch3/1  "<u_rate_yaw>"
  Bus Selector1/4 -> Mux/5  "<u_rate_roll>"
  Bus Selector1/5 -> Mux/6  "<u_rate_pitch>"
  Constant2/1 -> Mux/1
  Constant3/1 -> Logical Operator/3
  Switch12/1 -> Mux1/2, Mux/2
  K/1 -> Mux1/3, Mux/3
  Switch6/1 -> Mux/8
  Subsystem/1(Out1) -> Logical Operator/1
  Constant4/1 -> Mux1/1
  Switch4/1 -> [sim_CarSend6]
  Mux1/1 -> Switch4/3
  Mux/1 -> Switch5/1
  Switch5/1 -> [carSend6]
  [sim_flag] -> Switch5/2, Switch4/2
  uav6/1 -> Switch6/3
  [mode1] -> Switch6/2, Switch6/1

== system SIMULINK_PID_Tracking/send_ctrl_signal_car1/Send Command 7 ==
  pos : Inport
  u : Inport  Port=2
  Bus Selector : BusSelector  OutputSignals=x,y  OutputAsBus=on
  Bus Selector1 : BusSelector  OutputSignals=u_vx,u_vy,u_vz,u_rate_roll,u_rate_pitch,u_rate_yaw
  Clock : Clock
  Compare To Constant : simulink/Logic and Bit Operations/Compare To Constant  relop=>=  const=0.1  OutDataTypeStr=boolean
  Constant : Constant  Value=sim_end_time
  Constant1 : Constant  Value=0
  Constant2 : Constant  Value=uav7num
  Constant3 : Constant  Value=Vel_Switch_17
  Constant4 : Constant  Value=0
  K : Gain
  K1 : Gain
  K2 : Gain
  Logical Operator : Logic  Inputs=3  AllPortsSameDT=off  OutDataTypeStr=boolean
  Mux : Mux  Inputs=8
  Mux1 : Mux  Inputs=5
  Subsystem : Subsystem
  Sum : Sum  Inputs=|-+
  Switch{1..3,6,12} (5 alike) : Switch  Criteria=u2 > Threshold  Threshold=0.001  SaturateOnIntegerOverflow=off  InputSameDT=off
  Switch4 : Switch  Criteria=u2 > Threshold  SaturateOnIntegerOverflow=off  InputSameDT=off
  Switch5 : Switch  Criteria=u2 > Threshold  SaturateOnIntegerOverflow=off  InputSameDT=off
  uav7 : Constant
  tag scope: carSend7=global, sim_CarSend7=global
  wires:
  Constant1/1 -> Switch3/3, Switch2/3, Switch1/3, Switch12/3
  K1/1 -> Mux1/5, Mux/7
  Switch1/1 -> K/1
  Bus Selector1/2 -> Switch1/1  "<u_vy>"
  Switch2/1 -> K2/1
  Bus Selector1/3 -> Switch2/1  "<u_vz>"
  Switch3/1 -> K1/1
  Logical Operator/1 -> Switch1/2, Switch12/2, Switch2/2, Switch3/2
  K2/1 -> Mux1/4, Mux/4
  Clock/1 -> Sum/1
  Constant/1 -> Sum/2
  Sum/1 -> Compare To Constant/1
  Compare To Constant/1 -> Logical Operator/2
  pos/1 -> Bus Selector/1
  Bus Selector/1 -> Subsystem/1(In1)
  u/1 -> Bus Selector1/1
  Bus Selector1/1 -> Switch12/1  "<u_vx>"
  Bus Selector1/6 -> Switch3/1  "<u_rate_yaw>"
  Bus Selector1/4 -> Mux/5  "<u_rate_roll>"
  Bus Selector1/5 -> Mux/6  "<u_rate_pitch>"
  Constant2/1 -> Mux/1
  Constant3/1 -> Logical Operator/3
  Switch12/1 -> Mux1/2, Mux/2
  K/1 -> Mux1/3, Mux/3
  Switch6/1 -> Mux/8
  Subsystem/1(Out1) -> Logical Operator/1
  Constant4/1 -> Mux1/1
  Switch4/1 -> [sim_CarSend7]
  Mux1/1 -> Switch4/3
  Mux/1 -> Switch5/1
  Switch5/1 -> [carSend7]
  [sim_flag] -> Switch5/2, Switch4/2
  uav7/1 -> Switch6/3
  [mode1] -> Switch6/2, Switch6/1

== system SIMULINK_PID_Tracking/send_ctrl_signal_car1/Send Command 8 ==
  pos : Inport
  u : Inport  Port=2
  Bus Selector : BusSelector  OutputSignals=x,y  OutputAsBus=on
  Bus Selector1 : BusSelector  OutputSignals=u_vx,u_vy,u_vz,u_rate_roll,u_rate_pitch,u_rate_yaw
  Clock : Clock
  Compare To Constant : simulink/Logic and Bit Operations/Compare To Constant  relop=>=  const=0.1  OutDataTypeStr=boolean
  Constant : Constant  Value=sim_end_time
  Constant1 : Constant  Value=0
  Constant2 : Constant  Value=uav8num
  Constant3 : Constant  Value=Vel_Switch_18
  Constant4 : Constant  Value=0
  K : Gain
  K1 : Gain
  K2 : Gain
  Logical Operator : Logic  Inputs=3  AllPortsSameDT=off  OutDataTypeStr=boolean
  Mux : Mux  Inputs=8
  Mux1 : Mux  Inputs=5
  Subsystem : Subsystem
  Sum : Sum  Inputs=|-+
  Switch{1..3,6,12} (5 alike) : Switch  Criteria=u2 > Threshold  Threshold=0.001  SaturateOnIntegerOverflow=off  InputSameDT=off
  Switch4 : Switch  Criteria=u2 > Threshold  SaturateOnIntegerOverflow=off  InputSameDT=off
  Switch5 : Switch  Criteria=u2 > Threshold  SaturateOnIntegerOverflow=off  InputSameDT=off
  uav8 : Constant
  tag scope: carSend8=global, sim_CarSend8=global
  wires:
  Constant1/1 -> Switch3/3, Switch2/3, Switch1/3, Switch12/3
  K1/1 -> Mux1/5, Mux/7
  Switch1/1 -> K/1
  Bus Selector1/2 -> Switch1/1  "<u_vy>"
  Switch2/1 -> K2/1
  Bus Selector1/3 -> Switch2/1  "<u_vz>"
  Switch3/1 -> K1/1
  Logical Operator/1 -> Switch1/2, Switch12/2, Switch2/2, Switch3/2
  K2/1 -> Mux1/4, Mux/4
  Clock/1 -> Sum/1
  Constant/1 -> Sum/2
  Sum/1 -> Compare To Constant/1
  Compare To Constant/1 -> Logical Operator/2
  pos/1 -> Bus Selector/1
  Bus Selector/1 -> Subsystem/1(In1)
  u/1 -> Bus Selector1/1
  Bus Selector1/1 -> Switch12/1  "<u_vx>"
  Bus Selector1/6 -> Switch3/1  "<u_rate_yaw>"
  Bus Selector1/4 -> Mux/5  "<u_rate_roll>"
  Bus Selector1/5 -> Mux/6  "<u_rate_pitch>"
  Constant2/1 -> Mux/1
  Constant3/1 -> Logical Operator/3
  Switch12/1 -> Mux1/2, Mux/2
  K/1 -> Mux1/3, Mux/3
  Switch6/1 -> Mux/8
  Subsystem/1(Out1) -> Logical Operator/1
  Constant4/1 -> Mux1/1
  Switch4/1 -> [sim_CarSend8]
  Mux1/1 -> Switch4/3
  Mux/1 -> Switch5/1
  Switch5/1 -> [carSend8]
  [sim_flag] -> Switch5/2, Switch4/2
  uav8/1 -> Switch6/3
  [mode1] -> Switch6/2, Switch6/1

== system SIMULINK_PID_Tracking/send_ctrl_signal_car1/Send Command 9 ==
  pos : Inport
  u : Inport  Port=2
  Bus Selector : BusSelector  OutputSignals=x,y  OutputAsBus=on
  Bus Selector1 : BusSelector  OutputSignals=u_vx,u_vy,u_vz,u_rate_roll,u_rate_pitch,u_rate_yaw
  Clock : Clock
  Compare To Constant : simulink/Logic and Bit Operations/Compare To Constant  relop=>=  const=0.1  OutDataTypeStr=boolean
  Constant : Constant  Value=sim_end_time
  Constant1 : Constant  Value=0
  Constant2 : Constant  Value=uav9num
  Constant3 : Constant  Value=Vel_Switch_19
  Constant4 : Constant  Value=0
  K : Gain
  K1 : Gain
  K2 : Gain
  Logical Operator : Logic  Inputs=3  AllPortsSameDT=off  OutDataTypeStr=boolean
  Mux : Mux  Inputs=8
  Mux1 : Mux  Inputs=5
  Subsystem : Subsystem
  Sum : Sum  Inputs=|-+
  Switch{1..3,6,12} (5 alike) : Switch  Criteria=u2 > Threshold  Threshold=0.001  SaturateOnIntegerOverflow=off  InputSameDT=off
  Switch4 : Switch  Criteria=u2 > Threshold  SaturateOnIntegerOverflow=off  InputSameDT=off
  Switch5 : Switch  Criteria=u2 > Threshold  SaturateOnIntegerOverflow=off  InputSameDT=off
  uav9 : Constant
  tag scope: carSend9=global, sim_CarSend9=global
  wires:
  Constant1/1 -> Switch3/3, Switch2/3, Switch1/3, Switch12/3
  K1/1 -> Mux1/5, Mux/7
  Switch1/1 -> K/1
  Bus Selector1/2 -> Switch1/1  "<u_vy>"
  Switch2/1 -> K2/1
  Bus Selector1/3 -> Switch2/1  "<u_vz>"
  Switch3/1 -> K1/1
  Logical Operator/1 -> Switch1/2, Switch12/2, Switch2/2, Switch3/2
  K2/1 -> Mux1/4, Mux/4
  Clock/1 -> Sum/1
  Constant/1 -> Sum/2
  Sum/1 -> Compare To Constant/1
  Compare To Constant/1 -> Logical Operator/2
  pos/1 -> Bus Selector/1
  Bus Selector/1 -> Subsystem/1(In1)
  u/1 -> Bus Selector1/1
  Bus Selector1/1 -> Switch12/1  "<u_vx>"
  Bus Selector1/6 -> Switch3/1  "<u_rate_yaw>"
  Bus Selector1/4 -> Mux/5  "<u_rate_roll>"
  Bus Selector1/5 -> Mux/6  "<u_rate_pitch>"
  Constant2/1 -> Mux/1
  Constant3/1 -> Logical Operator/3
  Switch12/1 -> Mux1/2, Mux/2
  K/1 -> Mux1/3, Mux/3
  Switch6/1 -> Mux/8
  Subsystem/1(Out1) -> Logical Operator/1
  Constant4/1 -> Mux1/1
  Switch4/1 -> [sim_CarSend9]
  Mux1/1 -> Switch4/3
  Mux/1 -> Switch5/1
  Switch5/1 -> [carSend9]
  [sim_flag] -> Switch5/2, Switch4/2
  uav9/1 -> Switch6/3
  [mode1] -> Switch6/2, Switch6/1

== system SIMULINK_PID_Tracking/send_ctrl_signal_car1/Subsystem ==
  states_d : Inport
  ctrl : Inport  Port=2
  Bus Selector : BusSelector  OutputSignals=statesCAR1_2_d,statesCAR3_4_d,statesCAR5_6_d,statesCAR7_8_d,statesCAR9_10_d
  Bus Selector1 : BusSelector  OutputSignals=droneyeeCAR1_states,droneyeeCAR2_states  OutputAsBus=on
  Bus Selector2 : BusSelector  OutputSignals=ctrlCAR1_2,ctrlCAR3_4,ctrlCAR5_6,ctrlCAR7_8,ctrlCAR9_10
  Bus Selector5 : BusSelector  OutputSignals=droneyeeCAR9_states,droneyeeCAR10_states  OutputAsBus=on
  Bus Selector6 : BusSelector  OutputSignals=droneyeeCAR3_states,droneyeeCAR4_states  OutputAsBus=on
  Bus Selector7 : BusSelector  OutputSignals=droneyeeCAR5_states,droneyeeCAR6_states  OutputAsBus=on
  Bus Selector8 : BusSelector  OutputSignals=droneyeeCAR7_states,droneyeeCAR8_states  OutputAsBus=on
  logger_UAV : Subsystem
  wires:
  Bus Selector/1 -> logger_UAV/6(state_d1_2)  "<statesCAR1_2_d>"
  Bus Selector/2 -> logger_UAV/7(state_d3_4)  "<statesCAR3_4_d>"
  [uav_states] -> Bus Selector8/1, Bus Selector7/1, Bus Selector6/1, Bus Selector1/1, Bus Selector5/1
  Bus Selector1/1 -> logger_UAV/1(state1_2)
  Bus Selector6/1 -> logger_UAV/2(state3_4)
  Bus Selector2/2 -> logger_UAV/12(u3_4)  "<ctrlCAR3_4>"
  Bus Selector2/1 -> logger_UAV/11(u1_2)  "<ctrlCAR1_2>"
  Bus Selector7/1 -> logger_UAV/3(state5_6)
  Bus Selector2/3 -> logger_UAV/13(u5_6)  "<ctrlCAR5_6>"
  states_d/1 -> Bus Selector/1
  ctrl/1 -> Bus Selector2/1
  Bus Selector/3 -> logger_UAV/8(state_d5_6)  "<statesCAR5_6_d>"
  Bus Selector8/1 -> logger_UAV/4(state7_8)
  Bus Selector5/1 -> logger_UAV/5(In5)
  Bus Selector/4 -> logger_UAV/9(In9)  "<statesCAR7_8_d>"
  Bus Selector/5 -> logger_UAV/10(In10)  "<statesCAR9_10_d>"
  Bus Selector2/4 -> logger_UAV/14(In14)  "<ctrlCAR7_8>"
  Bus Selector2/5 -> logger_UAV/15(In15)  "<ctrlCAR9_10>"

== system SIMULINK_PID_Tracking/CMD_UAV/CMD1/Subsystem ==
  clock : Inport
  uavstates : Inport  Port=2
  Constant : Constant  Value=uav1num
  Constant1 : Constant  Value=ys
  MATLAB Function : MATLAB Function  TreatAsAtomicUnit=on
  轨迹 : Constant
  避障 : Constant
  队形 : Constant
  "xd " : Outport  VectorParamsAs1DForOutWhenUnconnected=off
  yd : Outport  Port=2  VectorParamsAs1DForOutWhenUnconnected=off
  zd : Outport  Port=3  VectorParamsAs1DForOutWhenUnconnected=off
  tag scope: avo_flag=global, form_flag=global, trj_flag=global
  wires:
  MATLAB Function/1(x_) -> "xd "/1
  MATLAB Function/2(y_) -> yd/1
  MATLAB Function/3(z_) -> zd/1
  clock/1 -> MATLAB Function/1(timestamp)
  Constant/1 -> MATLAB Function/2(uavnum)
  [switch_flag] -> MATLAB Function/3(switch_flag)
  uavstates/1 -> MATLAB Function/4(stas)
  轨迹/1 -> [trj_flag]
  队形/1 -> [form_flag]
  避障/1 -> [avo_flag]
  [trj_flag] -> MATLAB Function/5(trj_flag)
  [form_flag] -> MATLAB Function/6(form_flag)
  [avo_flag] -> MATLAB Function/7(avo_flag)
  Constant1/1 -> MATLAB Function/8(ref)

== system SIMULINK_PID_Tracking/CMD_UAV/CMD10/Subsystem ==
  clock : Inport
  uavstates : Inport  Port=2
  Constant : Constant  Value=uav10num
  Goto : Goto  Commented=on  GotoTag=trj_flag  TagVisibility=global
  Goto1 : Goto  Commented=on  GotoTag=form_flag  TagVisibility=global
  Goto2 : Goto  Commented=on  GotoTag=avo_flag  TagVisibility=global
  MATLAB Function : MATLAB Function  TreatAsAtomicUnit=on
  轨迹 : Constant  Commented=on
  避障 : Constant  Commented=on  Value=0
  队形 : Constant  Commented=on
  "xd " : Outport  VectorParamsAs1DForOutWhenUnconnected=off
  yd : Outport  Port=2  VectorParamsAs1DForOutWhenUnconnected=off
  zd : Outport  Port=3  VectorParamsAs1DForOutWhenUnconnected=off
  wires:
  MATLAB Function/1(x_) -> "xd "/1
  MATLAB Function/2(y_) -> yd/1
  MATLAB Function/3(z_) -> zd/1
  clock/1 -> MATLAB Function/1(timestamp)
  Constant/1 -> MATLAB Function/2(uavnum)
  [switch_flag] -> MATLAB Function/3(switch_flag)
  uavstates/1 -> MATLAB Function/4(stas)
  轨迹/1 -> Goto/1
  队形/1 -> Goto1/1
  避障/1 -> Goto2/1
  [trj_flag] -> MATLAB Function/5(trj_flag)
  [form_flag] -> MATLAB Function/6(form_flag)
  [avo_flag] -> MATLAB Function/7(avo_flag)

== system SIMULINK_PID_Tracking/CMD_UAV/CMD2/Subsystem ==
  clock : Inport
  uavstates : Inport  Port=2
  Constant : Constant  Value=uav2num
  MATLAB Function : MATLAB Function  TreatAsAtomicUnit=on
  "xd " : Outport  VectorParamsAs1DForOutWhenUnconnected=off
  yd : Outport  Port=2  VectorParamsAs1DForOutWhenUnconnected=off
  zd : Outport  Port=3  VectorParamsAs1DForOutWhenUnconnected=off
  wires:
  uavstates/1 -> MATLAB Function/4(stas)
  [switch_flag] -> MATLAB Function/3(switch_flag)
  [avo_flag] -> MATLAB Function/7(avo_flag)
  [trj_flag] -> MATLAB Function/5(trj_flag)
  Constant/1 -> MATLAB Function/2(uavnum)
  [form_flag] -> MATLAB Function/6(form_flag)
  clock/1 -> MATLAB Function/1(timestamp)
  MATLAB Function/1(x_) -> "xd "/1
  MATLAB Function/3(z_) -> zd/1
  MATLAB Function/2(y_) -> yd/1
